simulink model "task3"  (R2024a)
settings: Solver=VariableStepAuto  StartTime=0.0  StopTime=10.0  MaxStep=0.001  RelTol=1e-3
undefined symbols (not defined in the file): Abar, Bbar, Bfbar, C, D, Df, Gamma_f, K, wf0, x0_bar, Yf
settings Model: Creator=sizgr  LastModifiedBy=sizgr

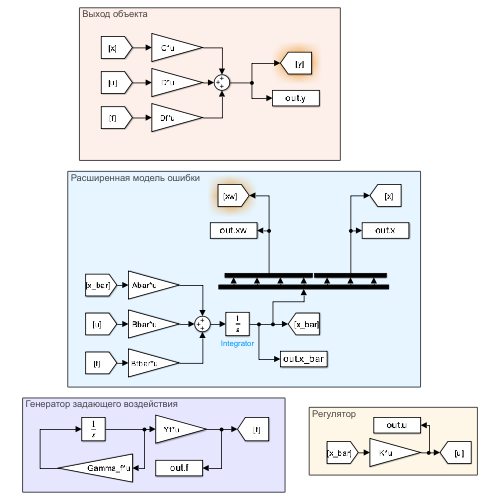
[thumbnail: Simulink's stored preview of the top-level diagram]
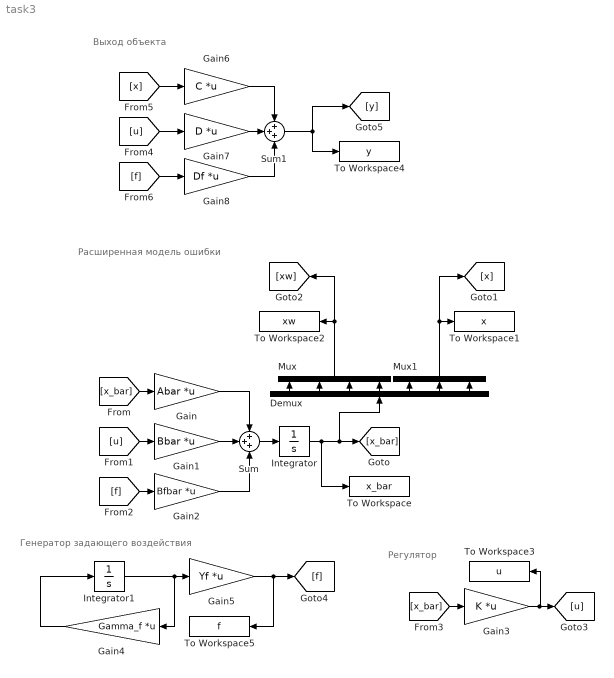
== system task3 ==
  note: Выход объекта
  note: Генератор задающего воздействия
  note: Регулятор
  note: Расширенная модель ошибки
  Demux : Demux  Outputs=7
  Gain : Gain  Gain=Abar  Multiplication=Matrix(K*u)
  Gain1 : Gain  Gain=Bbar  Multiplication=Matrix(K*u)
  Gain2 : Gain  Gain=Bfbar  Multiplication=Matrix(K*u)
  Gain3 : Gain  Gain=K  Multiplication=Matrix(K*u)
  Gain4 : Gain  Gain=Gamma_f  Multiplication=Matrix(K*u)
  Gain5 : Gain  Gain=Yf  Multiplication=Matrix(K*u)
  Gain6 : Gain  Gain=C  Multiplication=Matrix(K*u)
  Gain7 : Gain  Gain=D  Multiplication=Matrix(K*u)
  Gain8 : Gain  Gain=Df  Multiplication=Matrix(K*u)
  Integrator : Integrator  InitialCondition=x0_bar
  Integrator1 : Integrator  InitialCondition=wf0
  Mux : Mux
  Mux1 : Mux  Inputs=3
  Sum : Sum  Inputs=+++
  Sum1 : Sum  Inputs=+++
  To Workspace : ToWorkspace  VariableName=x_bar  SaveFormat=Timeseries  SampleTime=-1
  To Workspace1 : ToWorkspace  VariableName=x  SaveFormat=Timeseries  SampleTime=-1
  To Workspace2 : ToWorkspace  VariableName=xw  SaveFormat=Timeseries  SampleTime=-1
  To Workspace3 : ToWorkspace  VariableName=u  SaveFormat=Timeseries  SampleTime=-1
  To Workspace4 : ToWorkspace  VariableName=y  SaveFormat=Timeseries  SampleTime=-1
  To Workspace5 : ToWorkspace  VariableName=f  SaveFormat=Timeseries  SampleTime=-1
  wires:
  Sum/1 -> Integrator/1
  Integrator/1 -> Demux/1, [x_bar], To Workspace/1
  [x_bar] -> Gain/1
  [u] -> Gain1/1
  [f] -> Gain2/1
  Gain1/1 -> Sum/2
  Gain/1 -> Sum/1
  Gain2/1 -> Sum/3
  [x_bar] -> Gain3/1
  Gain3/1 -> To Workspace3/1, [u]
  Integrator1/1 -> Gain5/1, Gain4/1
  Gain4/1 -> Integrator1/1
  Gain5/1 -> [f], To Workspace5/1
  Gain6/1 -> Sum1/1
  Gain7/1 -> Sum1/2
  [u] -> Gain7/1
  [x] -> Gain6/1
  Sum1/1 -> To Workspace4/1, [y]
  [f] -> Gain8/1
  Gain8/1 -> Sum1/3
  Demux/1 -> Mux/1
  Demux/2 -> Mux/2
  Demux/3 -> Mux/3
  Mux/1 -> To Workspace2/1, [xw]
  Mux1/1 -> [x], To Workspace1/1
  Demux/5 -> Mux1/1
  Demux/6 -> Mux1/2
  Demux/7 -> Mux1/3
  Demux/4 -> Mux/4
